simulink model "sm_car"  (R2024a)
settings: Solver=ode23t  StartTime=0.0  StopTime=25  MaxStep=0.4  RelTol=1e-3  AbsTol=1e-3  EnableMultiTasking=on
PreLoadFcn:
  | % Due to usability issue in Repeating Sequence block
  | warning('off','Simulink:Masking:Invalid');
  | 
  | % Eliminate unnecessary warnings in inactive variants
  | % Warnings generated only if you click through inactive variant
  | warning('off','MATLAB:nonExistentField');
  | warning('off','Simulink:Parameters:BlkParamUndefined');
PostLoadFcn:
  | set_param([bdroot '/Vehicle'],'popup_trailer','Off')
  | warning('off','sm:sli:setup:compile:LocalSolverNotSupported')
  | %sm_car_config_maneuver(bdroot,'WOT Braking');
  | sm_car_config_vehicle(bdroot,'false');
  | sm_car_config_logging(bdroot);
InitFcn:
  | sm_car_config_camera;
  | Vehicle = sm_car_vehcfg_checkConfig(Vehicle);
  | sm_car_check_tire_model(bdroot);
StartFcn:
  | tic;
StopFcn:
  | Elapsed_Sim_Time = toc;
  | % disp(['Elapsed Sim Time = ' num2str(Elapsed_Sim_Time)]);
values from neighbouring files (symbols this model uses):
  EFFECTIVE_ROLLING_RADIUS_OF_TIRES_M = 0.23323    [vehicle_specs.m]
  MAXIMUM_CONTINUOUS_CURRENT_DRAW_A = 200    [vehicle_specs.m]
  MAXIMUM_NEGATIVE_TORQUE_FROM_MOTOR_Nm = -250    [vehicle_specs.m]
  MAXIMUM_TORQUE_FROM_MOTOR_Nm = 250    [vehicle_specs.m]
  TARGET_SLIP_RATIO = 0.10    (= 0.1)    [vehicle_specs.m]
undefined symbols (not defined in the file or in its folder): Axle1D, AxleIn, Camera, Control, Driver, Init, Maneuver, Pedal, RaceFix, RaceSpin, Scene, ShaftL1, ShaftL2, ShaftR1, ShaftR2, Visual, X, xy_data_car_side, Y, Z
libraries: sm_lib x1112, nesl_utility x285, fl_lib x221, simulink x24, sdl_lib x16, SimscapeFluids_lib x9, ee_lib x5, Linkage_Systems x4, Tire_1x2x x4, simulink_extras x3, slpidlib x2, AntiRollBar_Systems x2
(part 43 of 43)

== stateflow chart sm_car/Controller/TrqVec 4Motor/Brake Control/ABS/Valve Control L2/Logic ==
  state Inactive
    entry:
    Mod_State = 1;
    Mod_Dur = 10;
  state Initial_Release
    entry:
    Mod_State = 2;
    Mod_Dur = 10;
  state Initial_Apply
    entry:
    Mod_State = 1;
    Mod_Dur = 6;
  state Release
    entry:
    Mod_State = 2;
    Mod_Dur = 6;
  state Apply
    entry:
    Mod_State = 1;
    Mod_Dur = 2;
  state Hold
    entry:
    Mod_State = 0;
    Mod_Dur = 6;
  (default) -> Inactive
  Apply -> Inactive [order 2] : [vSpdEst <0.1]
  Release -> Inactive [order 2] : [vSpdEst <0.1]
  Inactive -> Initial_Release : [Slip>0.5]
  Initial_Release -> Initial_Apply : [Slip<0.1]
  Release -> Initial_Apply [order 1] : [Slip <0.05]
  Initial_Apply -> Hold [order 2] : [Slip>0.1]
  Initial_Apply -> Apply [order 1] : [after(10,msec)]
  Hold -> Release [order 2] : [Slip > 0.25]
  Hold -> Apply [order 1] : [after(40,msec)]
  Apply -> Hold [order 1] : [Slip > 0.1]
  data: Slip input; Mod_State output; Mod_Dur output; vSpdEst input

== stateflow chart sm_car/Controller/TrqVec 4Motor/Brake Control/ABS/Valve Control R1/Logic ==
  state Inactive
    entry:
    Mod_State = 1;
    Mod_Dur = 10;
  state Initial_Release
    entry:
    Mod_State = 2;
    Mod_Dur = 10;
  state Initial_Apply
    entry:
    Mod_State = 1;
    Mod_Dur = 6;
  state Release
    entry:
    Mod_State = 2;
    Mod_Dur = 6;
  state Apply
    entry:
    Mod_State = 1;
    Mod_Dur = 2;
  state Hold
    entry:
    Mod_State = 0;
    Mod_Dur = 6;
  (default) -> Inactive
  Apply -> Inactive [order 2] : [vSpdEst <0.1]
  Release -> Inactive [order 2] : [vSpdEst <0.1]
  Inactive -> Initial_Release : [Slip>0.5]
  Initial_Release -> Initial_Apply : [Slip<0.1]
  Release -> Initial_Apply [order 1] : [Slip <0.05]
  Initial_Apply -> Hold [order 2] : [Slip>0.1]
  Initial_Apply -> Apply [order 1] : [after(10,msec)]
  Hold -> Release [order 2] : [Slip > 0.25]
  Hold -> Apply [order 1] : [after(40,msec)]
  Apply -> Hold [order 1] : [Slip > 0.1]
  data: Slip input; Mod_State output; Mod_Dur output; vSpdEst input

== stateflow chart sm_car/Controller/TrqVec 4Motor/Brake Control/ABS/Valve Control R2/Logic ==
  state Inactive
    entry:
    Mod_State = 1;
    Mod_Dur = 10;
  state Initial_Release
    entry:
    Mod_State = 2;
    Mod_Dur = 10;
  state Initial_Apply
    entry:
    Mod_State = 1;
    Mod_Dur = 6;
  state Release
    entry:
    Mod_State = 2;
    Mod_Dur = 6;
  state Apply
    entry:
    Mod_State = 1;
    Mod_Dur = 2;
  state Hold
    entry:
    Mod_State = 0;
    Mod_Dur = 6;
  (default) -> Inactive
  Apply -> Inactive [order 2] : [vSpdEst <0.1]
  Release -> Inactive [order 2] : [vSpdEst <0.1]
  Inactive -> Initial_Release : [Slip>0.5]
  Initial_Release -> Initial_Apply : [Slip<0.1]
  Release -> Initial_Apply [order 1] : [Slip <0.05]
  Initial_Apply -> Hold [order 2] : [Slip>0.1]
  Initial_Apply -> Apply [order 1] : [after(10,msec)]
  Hold -> Release [order 2] : [Slip > 0.25]
  Hold -> Apply [order 1] : [after(40,msec)]
  Apply -> Hold [order 1] : [Slip > 0.1]
  data: Slip input; Mod_State output; Mod_Dur output; vSpdEst input

== matlab function sm_car/Driver/Closed Loop/Maneuver/MATLAB Function ==
  data: ad output; ref_z output; ref_x output; ref_y output; ref_ayaw output; vTarget output; cp output; p input; q input; posx input; posy input; posz input; xywin input; speed input; yaw input; dist input; pd input; maxld input; minSpd input; speedGain input; ld output; idx_ptMin output; simres output; idx_ptMin_prev input
function [ad,ref_z,ref_x,ref_y,ref_ayaw,vTarget,cp,ld, idx_ptMin, simres] = getPoseCurRef(p,q,posx,posy,posz,xywin,speed,yaw,dist,pd, maxld, minSpd, speedGain, idx_ptMin_prev)

% This function determines the target pose for the vehicle.  It
% interpolates within the provided trajectory to determine the target
% x-y position, yaw angle, and speed. The targets are defined with respect
% to distance along the target trajectory.  The first portion of the
% function determines the distance along the trajectory that the vehicle
% has traveled (ad).  Once that is found, the function interpolates to find
% the target pose at the preview distance (ad+pd).

npts = length(posx);

% Look for nearest point in a window near last evaluation
% Obtain window
if (idx_ptMin_prev == -1)
    % For first evaluation, use entire list of points
    ptlist = 1:npts;
elseif((idx_ptMin_prev-xywin)<1)
    % Window overlaps at lower end: take points from upper end
    win2 = (npts+idx_ptMin_prev-xywin):1:npts;
    win1 = 1:(idx_ptMin_prev+xywin);
    ptlist = [win1 win2];
elseif((idx_ptMin_prev+xywin)>npts)
    % Window overlaps at upper end: take points from lower end
    win2 = (idx_ptMin_prev-xywin):1:npts;
    win1 = 1:(idx_ptMin_prev+xywin-npts);
    ptlist = [win1 win2];
else
    % No overlap: use window
    ptlist = (idx_ptMin_prev-xywin):1:(idx_ptMin_prev+xywin);
end

% Find closest supplied trajectory point to current car position
distances = hypot(p(1) - posx,p(2) - posy);
distances_srch = distances(ptlist);
[~, idx_ptlist] = min(distances_srch);
idx_ptMin = ptlist(idx_ptlist);

%% Identify two trajectory points ahead of and behind closest supplied point
% A, B, C (closest), D, E
idx_ptC = idx_ptMin;
idx_ptA = idx_ptMin-2;
idx_ptB = idx_ptMin-1;
idx_ptD = idx_ptMin+1;
idx_ptE = idx_ptMin+2;

% If we are at end of trajectory, wrap point index
if (idx_ptA<=0),   idx_ptA = idx_ptA+npts; end
if (idx_ptB<=0),   idx_ptB = idx_ptB+npts; end
if (idx_ptD>npts), idx_ptD = idx_ptD-npts; end
if (idx_ptE>npts), idx_ptE = idx_ptE-npts; end

% Extract trajectory point x-y locations
ptA = [posx(idx_ptA); posy(idx_ptA)];
ptB = [posx(idx_ptB); posy(idx_ptB)];
ptC = [posx(idx_ptC); posy(idx_ptC)];
ptD = [posx(idx_ptD); posy(idx_ptD)];
ptE = [posx(idx_ptE); posy(idx_ptE)];

%% Find line separating trajectory segments BC, CD
% Find angle of line connecting BD
qBD = atan2(ptD(2)-ptB(2),ptD(1)-ptB(1));

% Angle of line separating BC, CD is normal to that line
qC  = qBD+pi/2;

%% Determine if we are nearest to trajectory segment BC or BD
% Check if vehicle location and point B on same side of line
% separating segments BC and BD
segBC = arePointsOnSameSide(ptC(1), ptC(2), tan(qC), p(1), p(2), ptB(1), ptB(2));

%% Find vehicle line segment 
% Segment is parallel to closest trajectory segment on which vehicle lies
if(segBC)
   % Use segment BC
   % Line dividing segments AB and BC is normal to line AC 
   qR = atan2(ptC(2)-ptA(2),ptC(1)-ptA(1))+pi/2;
   % Line dividing segments BC and CD has already been found 
   qF = qC;

   ptR = ptB;  % Rear point of segment is point B
   ptF = ptC;  % Front point of segment is point C

   % Angle of vehicle line segment is same as angle of segment BC
   qV = atan2(ptC(2)-ptB(2),ptC(1)-ptB(1));
    % Distance along trajectory to rear of segment
   distR    = dist(idx_ptB);
else
   % Use segment CD
   % Line dividing segments BC and CD has already been found 
   qR = qC;
   % Line dividing segments CD and DE is normal to line CE 
   qF = atan2(ptE(2)-ptC(2),ptE(1)-ptC(1))+pi/2;

   ptR = ptC;    % Rear point of segment is point B
   ptF = ptD;    % Front point of segment is point C

   % Angle of vehicle line segment is same as angle of segment CD
   qV = atan2(ptD(2)-ptC(2),ptD(1)-ptC(1));
    % Distance along trajectory to rear of segment
   distR = dist(idx_ptC);
end

% Length of trajectory segment
distSeg  = sqrt((ptF(1)-ptR(1))^2+(ptF(2)-ptR(2))^2);

% Find endpoints of vehicle line segment
[xR, yR] = findIntersection(p(1), p(2), tan(qV), ptR(1), ptR(2), tan(qR));
[xF, yF] = findIntersection(p(1), p(2), tan(qV), ptF(1), ptF(2), tan(qF));

% Length of vehicle line segment
distFR = sqrt((xR-xF)^2+(yR-yF)^2);
% Distance of vehicle location from rear of vehicle line segment
distvR = sqrt((xR-p(1))^2+(yR-p(2))^2);

% Percentage of distance from vehicle to rear of vehicle line segment 
% Do not permit percentage to go above 100%
% Occurs when vehicle is far from line on inside of curve
segPcnt = min(distvR/distFR,1);

% Distance along trajectory = 
%   Distance to rear of trajectory segment + 
%   length of closest trajectory segment * 
%   percent of vehicle line segment already completed
ad = distR+segPcnt*distSeg;

% Find angle between vehicle location, forward point, and track trajectory
vec_F2v  = ptF - [p(1); p(2)];
vec_F2R  = ptF - ptR;

% Use cosine formula to obtain angle
cos_ang_new = dot(vec_F2v,vec_F2R)/(norm(vec_F2v)*norm(vec_F2R));

% Bound cosine of angle between eps and 1
cos_ang_new = max(cos_ang_new,eps);
cos_ang_new = min(cos_ang_new,1-eps);

% Use angle to obtain lateral distance of vehicle from trajectory
ld = norm(vec_F2v)*sin(acos(cos_ang_new));

% Pose targets for Stanley controller (distance cumulatively sums)
dist4interp = [-dist(end)+dist(1:end-1); dist; dist(end)+dist(2:end)];
posx4interp = [           posx(1:end-1); posx;           posx(2:end)];
posy4interp = [           posy(1:end-1); posy;           posy(2:end)];
posz4interp = [           posz(1:end-1); posz;           posz(2:end)];
speed4interp= [          speed(1:end-1);speed;          speed(2:end)];
% Wrap the interpolation vector for yaw.  
% Necessary to avoid obtaining values between yaw(end) and yaw(1)
yaw4interp  = [-(yaw(end)-yaw(1)) + yaw(1:end-1);  yaw;  (yaw(end)-yaw(1))+ yaw(2:end)];

% Current point
cp = [p(1);p(2);q(3)*180/pi]';

% Reference point obtained from supplied trajectory
% Interpolate using Actual distance (ad) + preview distance (pd)
ref_x    = interp1(dist4interp,posx4interp,ad+pd,'pchip');
ref_y    = interp1(dist4interp,posy4interp,ad+pd,'pchip');
ref_ayaw = interp1(dist4interp,yaw4interp, ad+pd,'pchip');

% For visualization only
ref_z    = interp1(dist4interp,posz4interp,ad+pd);

% Reference velocity obtained from supplied trajectory
% Interpolate using actual distance
vx_cp = interp1(dist4interp,speed4interp,ad);

% Protect for NaNs
ref_x(isnan(ref_x)) = 0;
ref_y(isnan(ref_y)) = 0;
ref_ayaw(isnan(ref_ayaw)) = 0;
ref_z(isnan(ref_z)) = 0;

% Scale speed target
% Reduce speed target if car is far from the target trajectory
if ld < maxld
    vTarget = vx_cp * speedGain;
else
    vTarget = minSpd;
end

% Outputs for debugging calculation
simres = [idx_ptA idx_ptB idx_ptC idx_ptD idx_ptE qC segBC segPcnt xR yR  xF yF p(1) p(2) ad distR distSeg];

end

function [x_intersect, y_intersect] = findIntersection(x1, y1, m1, x2, y2, m2)
    % Check if the slopes are equal (parallel lines)
    if m1 == m2
        error('Invalid trajectory points. The lines are parallel and do not intersect.');
    end
    
    % Calculate the intersection point
    x_intersect = (y2 - y1 + m1*x1 - m2*x2) / (m1 - m2);
    y_intersect = m1 * (x_intersect - x1) + y1;
end

function same_side = arePointsOnSameSide(x0, y0, m, x1, y1, x2, y2)
    % Calculate the line coefficients
    a = -m; % Coefficient of x
    b = 1;  % Coefficient of y
    c = m*x0 - y0; % Constant term
    
    % Calculate the line equation value for both points
    value1 = a*x1 + b*y1 + c;
    value2 = a*x2 + b*y2 + c;
    
    % Check if both values have the same sign
    same_side = (value1 * value2) > 0;
end

== matlab function sm_car/Controller/Default/Firmware Controller/Pedal Sensor Error Detection System/APPS Implausibility ==
  data: apps_1_percentage input; apps_signals_are_fucked output; apps_2_percentage input
function apps_signals_are_fucked = fcn(apps_1_percentage, apps_2_percentage)

persistent isConditionActive startTime

if isempty(isConditionActive)
    isConditionActive = false;
    startTime = 0;
end

% must be for more than some amount of time
if (abs(apps_1_percentage - apps_2_percentage) > IMPLAUSIBLE_APPS_DIFFERENCE)
    if ~isConditionActive
        startTime = tic;
        isConditionActive = true;
    elseif toc(startTime) > DURATION_OF_EVENT_TO_TRIGGER_IMPLAUSIBILITY
        apps_signals_are_fucked = 1;
    else
        apps_signals_are_fucked = 0;
    end
else
    isConditionActive = false;
    apps_signals_are_fucked = 0;
end

== matlab function sm_car/Controller/Default/Firmware Controller/Pedal Sensor Error Detection System/APPS 1 Out of Range ==
  data: sensor_voltage input; signal_out_of_range output
function signal_out_of_range = fcn(sensor_voltage)

persistent isConditionActive startTime

if isempty(isConditionActive)
    isConditionActive = false;
    startTime = 0;
end

% must be for more than some amount of time
if (sensor_voltage < APPS_1_LOWER_VOLTAGE) || (sensor_voltage > APPS_1_UPPER_VOLTAGE)
    if ~isConditionActive
        startTime = tic;
        isConditionActive = true;
    elseif toc(startTime) > DURATION_OF_EVENT_TO_TRIGGER_IMPLAUSIBILITY_S
        signal_out_of_range = 1;
    else
        signal_out_of_range = 0;
    end
else
    isConditionActive = false;
    signal_out_of_range = 0;
end

== matlab function sm_car/Controller/Default/Firmware Controller/Pedal Sensor Error Detection System/APPS 1 Disconnected ==
  data: sensor_voltage input; signal_disconnected output
function signal_disconnected = fcn(sensor_voltage)

persistent isConditionActive startTime

if isempty(isConditionActive)
    isConditionActive = false;
    startTime = 0;
end

% must be for more than some amount of time
if (sensor_voltage < MINIMUM_VOLTAGE_REQUIRED_FOR_SENSOR_TO_NOT_BE_DISCONNECTED_V)
    if ~isConditionActive
        startTime = tic;
        isConditionActive = true;
    elseif toc(startTime) > TIME_REQUIRED_FOR_SENSOR_TO_BE_DEEMED_DISCONNECTED_S
        signal_disconnected = 1;
    else
        signal_disconnected = 0;
    end
else
    isConditionActive = false;
    signal_disconnected = 0;
end

== matlab function sm_car/Controller/Default/Firmware Controller/Pedal Sensor Error Detection System/APPS 2 Disconnected ==
  data: sensor_voltage input; signal_disconnected output
function signal_disconnected = fcn(sensor_voltage)

persistent isConditionActive startTime

if isempty(isConditionActive)
    isConditionActive = false;
    startTime = 0;
end

% must be for more than some amount of time
if (sensor_voltage < MINIMUM_VOLTAGE_REQUIRED_FOR_SENSOR_TO_NOT_BE_DISCONNECTED_V)
    if ~isConditionActive
        startTime = tic;
        isConditionActive = true;
    elseif toc(startTime) > TIME_REQUIRED_FOR_SENSOR_TO_BE_DEEMED_DISCONNECTED_S
        signal_disconnected = 1;
    else
        signal_disconnected = 0;
    end
else
    isConditionActive = false;
    signal_disconnected = 0;
end

== matlab function sm_car/Controller/Default/Firmware Controller/Pedal Sensor Error Detection System/APPS 2 Out of Range ==
  data: sensor_voltage input; signal_out_of_range output
function signal_out_of_range = fcn(sensor_voltage)

persistent isConditionActive startTime

if isempty(isConditionActive)
    isConditionActive = false;
    startTime = 0;
end

% must be for more than some amount of time
if (sensor_voltage < APPS_1_LOWER_VOLTAGE) || (sensor_voltage > APPS_1_UPPER_VOLTAGE)
    if ~isConditionActive
        startTime = tic;
        isConditionActive = true;
    elseif toc(startTime) > DURATION_OF_EVENT_TO_TRIGGER_IMPLAUSIBILITY_S
        signal_out_of_range = 1;
    else
        signal_out_of_range = 0;
    end
else
    isConditionActive = false;
    signal_out_of_range = 0;
end

== matlab function sm_car/Controller/Default/Firmware Controller/Pedal Sensor Error Detection System/BSE Front Disconnected ==
  data: sensor_voltage input; signal_disconnected output
function signal_disconnected = fcn(sensor_voltage)

persistent isConditionActive startTime

if isempty(isConditionActive)
    isConditionActive = false;
    startTime = 0;
end

% must be for more than some amount of time
if (sensor_voltage < MINIMUM_VOLTAGE_REQUIRED_FOR_SENSOR_TO_NOT_BE_DISCONNECTED_V)
    if ~isConditionActive
        startTime = tic;
        isConditionActive = true;
    elseif toc(startTime) > TIME_REQUIRED_FOR_SENSOR_TO_BE_DEEMED_DISCONNECTED_S
        signal_disconnected = 1;
    else
        signal_disconnected = 0;
    end
else
    isConditionActive = false;
    signal_disconnected = 0;
end

== matlab function sm_car/Controller/Default/Firmware Controller/Pedal Sensor Error Detection System/BSE Front Out of Range ==
  data: sensor_voltage input; signal_out_of_range output
function signal_out_of_range = fcn(sensor_voltage)

persistent isConditionActive startTime

if isempty(isConditionActive)
    isConditionActive = false;
    startTime = 0;
end

% must be for more than some amount of time
if (sensor_voltage < BSE_FRONT_LOWER_VOLTAGE) || (sensor_voltage > BSE_FRONT_UPPER_VOLTAGE)
    if ~isConditionActive
        startTime = tic;
        isConditionActive = true;
    elseif toc(startTime) > DURATION_OF_EVENT_TO_TRIGGER_IMPLAUSIBILITY_S
        signal_out_of_range = 1;
    else
        signal_out_of_range = 0;
    end
else
    isConditionActive = false;
    signal_out_of_range = 0;
end

== matlab function sm_car/Controller/Default/Firmware Controller/Pedal Sensor Error Detection System/BSE Rear Disconnected ==
  data: sensor_voltage input; signal_disconnected output
function signal_disconnected = fcn(sensor_voltage)

persistent isConditionActive startTime

if isempty(isConditionActive)
    isConditionActive = false;
    startTime = 0;
end

% must be for more than some amount of time
if (sensor_voltage < MINIMUM_VOLTAGE_REQUIRED_FOR_SENSOR_TO_NOT_BE_DISCONNECTED_V)
    if ~isConditionActive
        startTime = tic;
        isConditionActive = true;
    elseif toc(startTime) > TIME_REQUIRED_FOR_SENSOR_TO_BE_DEEMED_DISCONNECTED_S
        signal_disconnected = 1;
    else
        signal_disconnected = 0;
    end
else
    isConditionActive = false;
    signal_disconnected = 0;
end

== matlab function sm_car/Controller/Default/Firmware Controller/Pedal Sensor Error Detection System/BSE Rear Out of Range ==
  data: sensor_voltage input; signal_out_of_range output
function signal_out_of_range = fcn(sensor_voltage)

persistent isConditionActive startTime

if isempty(isConditionActive)
    isConditionActive = false;
    startTime = 0;
end

% must be for more than some amount of time
if (sensor_voltage < BSE_REAR_LOWER_VOLTAGE) || (sensor_voltage > BSE_REAR_UPPER_VOLTAGE)
    if ~isConditionActive
        startTime = tic;
        isConditionActive = true;
    elseif toc(startTime) > DURATION_OF_EVENT_TO_TRIGGER_IMPLAUSIBILITY_S
        signal_out_of_range = 1;
    else
        signal_out_of_range = 0;
    end
else
    isConditionActive = false;
    signal_out_of_range = 0;
end

== matlab function sm_car/Controller/Default/Firmware Controller/Brakes are Engaged ==
  data: bse_front_percentage input; brakes_are_engaged output; bse_rear_percentage input
function brakes_are_engaged = fcn(bse_front_percentage, bse_rear_percentage)


if (bse_front_percentage > MINIMUM_BRAKE_THRESHOLD || bse_rear_percentage > MINIMUM_BRAKE_TRESHOLD)
    brakes_are_engaged = 1;
else
    brakes_are_engaged = 0;
end

== stateflow chart sm_car/Controller/Default/Firmware Controller/Chart ==
  state standby
  state buzzer
    entry:
    ready_to_drive_buzzer = 1;
    exit:
    ready_to_drive_buzzer = 0;
  state drive_enabled
    entry:
    motor_enabled = 1;
    exit:
    motor_enabled = 0;
  state both_accel_decel
  drive_enabled -> standby [order 6] : [bse_front_disconnected || bse_rear_disconnected]
  drive_enabled -> standby [order 5] : [apps_1_disconnected || apps_2_disconnected]
  (default) -> standby
  drive_enabled -> standby [order 4] : [bse_front_out_of_range || bse_rear_out_of_range]
  drive_enabled -> standby [order 3] : [apps_implausibility]
  drive_enabled -> standby [order 2] : [apps_1_out_of_range || apps_2_out_of_range]
  standby -> buzzer : [tractive_system_enabled && brakes_are_engaged && ignition_button_pressed]
  buzzer -> drive_enabled : [after(3,sec)]
  drive_enabled -> both_accel_decel [order 1] : [brakes_are_engaged && (apps_percentage > 0.25)]
  both_accel_decel -> drive_enabled : [apps_percentage < 0.05]
  data: brakes_are_engaged input; ignition_button_pressed input; tractive_system_enabled input; ready_to_drive_buzzer output; apps_1_disconnected input; apps_1_out_of_range input; apps_2_disconnected input; apps_2_out_of_range input; apps_implausibility input; apps_percentage input; bse_front_disconnected input; bse_front_out_of_range input; bse_rear_disconnected input; bse_rear_out_of_range input; motor_enabled output

== matlab function sm_car/Controller/Default/Firmware Controller/APPS 2 to Percentage ==
  data: apps_2_voltage input; apps_2_percentage output
function apps_2_percentage = convert_voltage_to_percentage(apps_2_voltage)

if (apps_2_voltage >= APPS_2_UPPER_VOLTAGE)  % if voltage is above maximum threshold, return 100.0
    apps_2_percentage = 100.0;
elseif (apps_2_voltage > APPS_2_LOWER_VOLTAGE)  
    apps_2_percentage = (apps_2_voltage - APPS_2_LOWER_VOLTAGE) / (APPS_2_UPPER_VOLTAGE - APPS_2_LOWER_VOLTAGE);
else  % if voltage is below minimum threshold, return 0
    apps_2_percentage = 0;
end

== matlab function sm_car/Controller/Default/Firmware Controller/APPS 1 to Percentage ==
  data: apps_1_voltage input; apps_1_percentage output
function apps_1_percentage = convert_voltage_to_percentage(apps_1_voltage)

if (apps_1_voltage >= APPS_1_UPPER_VOLTAGE)  % if voltage is above maximum threshold, return 100.0
    apps_1_percentage = 100.0;
elseif (apps_1_voltage > APPS_1_LOWER_VOLTAGE)  
    apps_1_percentage = (apps_1_voltage - APPS_1_LOWER_VOLTAGE) / (APPS_1_UPPER_VOLTAGE - APPS_1_LOWER_VOLTAGE);
else  % if voltage is below minimum threshold, return 0
    apps_1_percentage = 0;
end

== matlab function sm_car/Controller/Default/Firmware Controller/BSE Front to Percentage ==
  data: bse_front_voltage input; bse_front_percentage output
function bse_front_percentage = convert_voltage_to_percentage(bse_front_voltage)

if (bse_front_voltage >= BSE_FRONT_UPPER_VOLTAGE)  % if voltage is above maximum threshold, return 100.0
    bse_front_percentage = 100.0;
elseif (bse_front_voltage > BSE_FRONT_LOWER_VOLTAGE)  
    bse_front_percentage = (bse_front_voltage - BSE_FRONT_LOWER_VOLTAGE) / (BSE_FRONT_UPPER_VOLTAGE - BSE_FRONT_LOWER_VOLTAGE);
else  % if voltage is below minimum threshold, return 0
    bse_front_percentage = 0;
end

== matlab function sm_car/Controller/Default/Firmware Controller/BSE Rear to Percentage ==
  data: bse_rear_voltage input; bse_rear_percentage output
function bse_rear_percentage = convert_voltage_to_percentage(bse_rear_voltage)

if (bse_rear_voltage >= BSE_REAR_UPPER_VOLTAGE)  % if voltage is above maximum threshold, return 100.0
    bse_rear_percentage = 100.0;
elseif (bse_rear_voltage > BSE_REAR_LOWER_VOLTAGE)  
    bse_rear_percentage = (bse_rear_voltage - BSE_REAR_LOWER_VOLTAGE) / (BSE_REAR_UPPER_VOLTAGE - BSE_REAR_LOWER_VOLTAGE);
else  % if voltage is below minimum threshold, return 0
    bse_rear_percentage = 0;
end

== matlab function sm_car/Controller/TrqVec 4Motor/Power_TqVec/Torque Vectoring/Calculate Torque Split ==
  data: enable input; max_delta_trq input; max_tq input; tq_l_out output; tq_l input; tq_r input; tq_r_out output; tq_tv input; brk input
function [tq_l_out,tq_r_out] = fcn(enable,max_delta_trq,max_tq,tq_l,tq_r,tq_tv,brk)

% enable: flag to turn on torque vectoring
%         True if steering wheel is turned and non-zero vehicle speed
% brk   : flag to turn on torque vectoring
%         True if not braking


% Limit difference in torque between tires lower of 
% (input parameter) and max/min motor torque
t_lim=min(max_tq-abs(tq_l),max_tq-abs(tq_r));
delta_t=min(max_delta_trq,min(t_lim,abs(tq_tv)))*sign(tq_tv)*enable;

if brk>0 
    % Not braking. Use torque vectoring
    tq_l_out=(tq_l-delta_t)*brk;
    tq_r_out=(tq_r+delta_t)*brk;
else
    % No adjustments due to torque vectoring
    tq_l_out=tq_l;
    tq_r_out=tq_r;
end

== stateflow chart sm_car/Controller/TrqVec 4Motor/Brake Control/ABS/Valve Control L1/Logic ==
  state Inactive
    entry:
    Mod_State = 1;
    Mod_Dur = 10;
  state Initial_Release
    entry:
    Mod_State = 2;
    Mod_Dur = 10;
  state Initial_Apply
    entry:
    Mod_State = 1;
    Mod_Dur = 6;
  state Release
    entry:
    Mod_State = 2;
    Mod_Dur = 6;
  state Apply
    entry:
    Mod_State = 1;
    Mod_Dur = 2;
  state Hold
    entry:
    Mod_State = 0;
    Mod_Dur = 6;
  (default) -> Inactive
  Apply -> Inactive [order 2] : [vSpdEst <0.1]
  Release -> Inactive [order 2] : [vSpdEst <0.1]
  Inactive -> Initial_Release : [Slip>0.5]
  Initial_Release -> Initial_Apply : [Slip<0.1]
  Release -> Initial_Apply [order 1] : [Slip <0.05]
  Initial_Apply -> Hold [order 2] : [Slip>0.1]
  Initial_Apply -> Apply [order 1] : [after(10,msec)]
  Hold -> Release [order 2] : [Slip > 0.25]
  Hold -> Apply [order 1] : [after(40,msec)]
  Apply -> Hold [order 1] : [Slip > 0.1]
  data: Slip input; Mod_State output; Mod_Dur output; vSpdEst input
